simulink model "Lab8_model_nlin"  (R2017a)
settings: Solver=VariableStepAuto  StartTime=0.0  StopTime=10.0  RelTol=1e-3
values from neighbouring files (symbols this model uses):
  A = pi*R1*R1    (= 10.9999393421)    [Lab2.m]    (also in ModelDataNonlinear.m)
  a = (P1y - P2y) / (P1x - P2x)    (= 0.457251908397)    [Lab4.m]    (also in Lab8.m = 10; Lab9.m = 0.01)
  B = (pi*R2*R2)/(3*H2*H2)    (= 0.00337009933323)    [Lab2.m]    (also in Lab8.m = deltah20max / k; Lab9.m = 0.4; ModelDataNonlinear.m)
  C1 = 1.372    [Lab2.m]    (also in ModelDataNonlinear.m)
  C2 = 0.332756    [Lab2.m]    (also in ModelDataNonlinear.m)
  deltaw = deltaq1    [Lab2.m]    (also in Lab3.m = 0; Lab8.m = deltah20max / 3; ModelDataNonlinear.m = 0.1*w0)
  h10 = (q10/C1).^2    [Lab2.m]    (also in ModelDataNonlinear.m)
  h20 = h2max/2    (= 8)    [Lab2.m]    (also in ModelDataNonlinear.m)
  w0 = q10    [ModelDataNonlinear.m]
settings Model: Creator=ishiguro  LastModifiedBy=ishiguro

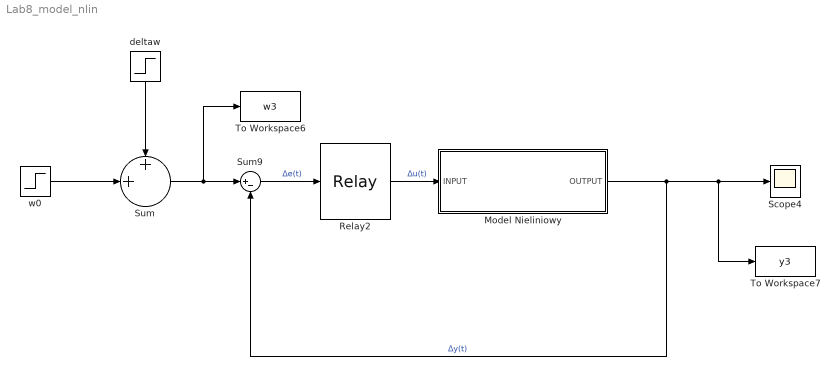
== system Lab8_model_nlin ==
  Model Nieliniowy : Subsystem
  Relay2 : Relay  OnSwitchValue=a  OffSwitchValue=a  OnOutputValue=B
  Scope4 : Scope
  Sum : Sum  Inputs=++|
  Sum9 : Sum  Inputs=|+-
  To Workspace6 : ToWorkspace  VariableName=w3  SaveFormat=Timeseries  SampleTime=-1
  To Workspace7 : ToWorkspace  VariableName=y3  SaveFormat=Timeseries  SampleTime=-1
  deltaw : Step  Time=0  After=deltaw  SampleTime=0
  "w0 " : Step  Time=0  After=w0  SampleTime=0
  wires:
  Sum/1 -> To Workspace6/1, Sum9/1
  Sum9/1 -> Relay2/1  "Δe(t)"
  deltaw/1 -> Sum/1
  Model Nieliniowy/1(OUTPUT) -> To Workspace7/1, Scope4/1, Sum9/2  "Δy(t)"
  Relay2/1 -> Model Nieliniowy/1(INPUT)  "Δu(t)"
  "w0 "/1 -> Sum/2

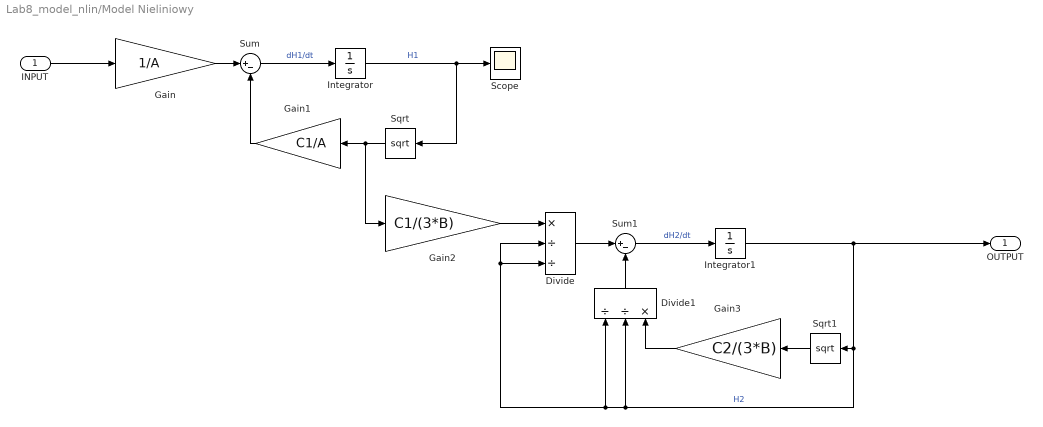
== system Lab8_model_nlin/Model Nieliniowy ==
  INPUT : Inport
  Divide : Product  Inputs=*//
  Divide1 : Product  Inputs=//*
  Gain : Gain  Gain=1/A
  Gain1 : Gain  Gain=C1/A
  Gain2 : Gain  Gain=C1/(3*B)
  Gain3 : Gain  Gain=C2/(3*B)
  Integrator : Integrator  InitialCondition=h10
  Integrator1 : Integrator  InitialCondition=h20  UpperSaturationLimit=999
  Scope : Scope
  Sqrt : Sqrt  SaturateOnIntegerOverflow=on
  Sqrt1 : Sqrt  SaturateOnIntegerOverflow=on
  Sum : Sum  Inputs=|+-
  Sum1 : Sum  Inputs=|+-
  OUTPUT : Outport
  wires:
  INPUT/1 -> Gain/1
  Sum/1 -> Integrator/1  "dH1/dt"
  Integrator/1 -> Sqrt/1, Scope/1  "H1"
  Sqrt/1 -> Gain2/1, Gain1/1
  Gain1/1 -> Sum/2
  Sum1/1 -> Integrator1/1  "dH2/dt"
  Sqrt1/1 -> Gain3/1
  Gain/1 -> Sum/1
  Gain3/1 -> Divide1/3
  Divide1/1 -> Sum1/2
  Divide/1 -> Sum1/1
  Gain2/1 -> Divide/1
  Integrator1/1 -> OUTPUT/1, Sqrt1/1, Divide1/2, Divide1/1, Divide/3, Divide/2  "H2"
